simulink model "Vjezba7"  (R2016b)
settings: Solver=FixedStepAuto  StartTime=0.0  StopTime=100  FixedStep=0.0001  RelTol=1e-3
libraries: simulink_extras x3, simulink x3
settings Model: Creator=Luka  LastModifiedBy=Luka

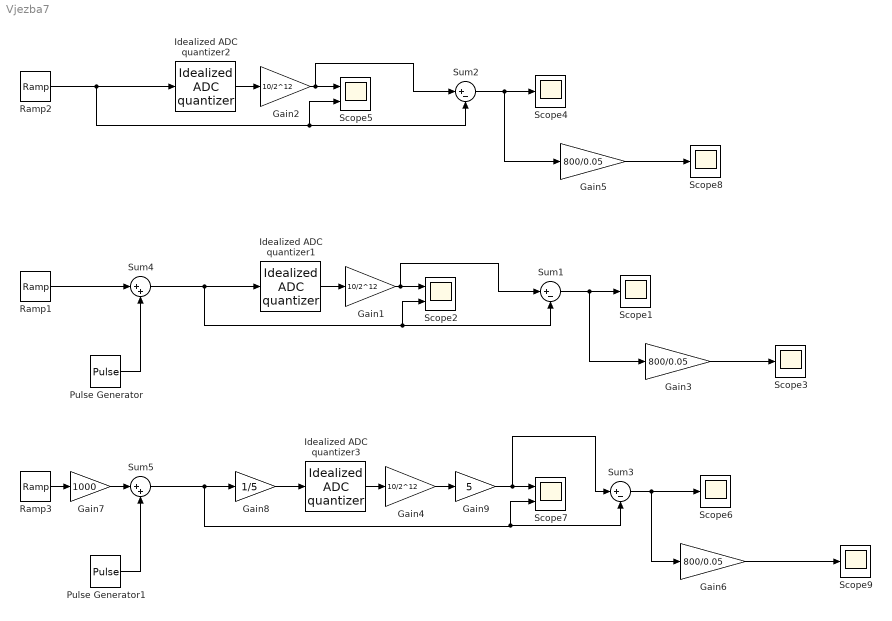
== system Vjezba7 ==
  Gain1 : Gain  Gain=10/2^12
  Gain2 : Gain  Gain=10/2^12
  Gain3 : Gain  Gain=800/0.05
  Gain4 : Gain  Gain=10/2^12
  Gain5 : Gain  Gain=800/0.05
  Gain6 : Gain  Gain=800/0.05
  Gain7 : Gain  Gain=1000
  Gain8 : Gain  Gain=1/5
  Gain9 : Gain  Gain=5
  Idealized ADC quantizer1 : simulink_extras/Additional Discrete/Idealized ADC quantizer  NumberOfConverterBits=12  Vmin=0  Vmax=10  OutputDataType=int16  OutputNegativeValues=off
  Idealized ADC quantizer2 : simulink_extras/Additional Discrete/Idealized ADC quantizer  NumberOfConverterBits=12  Vmin=0  Vmax=10  OutputDataType=int16  OutputNegativeValues=off
  Idealized ADC quantizer3 : simulink_extras/Additional Discrete/Idealized ADC quantizer  NumberOfConverterBits=12  Vmin=0  Vmax=10  OutputDataType=int16  OutputNegativeValues=off
  Pulse Generator : DiscretePulseGenerator  PulseType=Time based  Amplitude=0.01  Period=20  PulseWidth=3
  Pulse Generator1 : DiscretePulseGenerator  PulseType=Time based  Amplitude=0.01  Period=20  PulseWidth=3
  Ramp1 : simulink/Sources/Ramp  slope=0.05/800  start=0  X0=0
  Ramp2 : simulink/Sources/Ramp  slope=0.05/800  start=0  X0=0
  Ramp3 : simulink/Sources/Ramp  slope=0.05/800  start=0  X0=0
  Scope{1,3..4,6,8..9} (6 alike) : Scope
  Scope2 : Scope  NumInputPorts=2
  Scope5 : Scope  NumInputPorts=2
  Scope7 : Scope  NumInputPorts=2
  Sum1 : Sum  Inputs=|+-
  Sum2 : Sum  Inputs=|+-
  Sum3 : Sum  Inputs=|+-
  Sum4 : Sum  Inputs=|++
  Sum5 : Sum  Inputs=|++
  wires:
  Ramp2/1 -> Sum2/2, Scope5/2, Idealized ADC quantizer2/1
  Idealized ADC quantizer2/1 -> Gain2/1
  Gain2/1 -> Sum2/1, Scope5/1
  Sum2/1 -> Gain5/1, Scope4/1
  Gain5/1 -> Scope8/1
  Gain3/1 -> Scope3/1
  Sum1/1 -> Scope1/1, Gain3/1
  Gain1/1 -> Scope2/1, Sum1/1
  Idealized ADC quantizer1/1 -> Gain1/1
  Pulse Generator/1 -> Sum4/2
  Ramp1/1 -> Sum4/1
  Sum4/1 -> Scope2/2, Sum1/2, Idealized ADC quantizer1/1
  Pulse Generator1/1 -> Sum5/2
  Idealized ADC quantizer3/1 -> Gain4/1
  Sum3/1 -> Gain6/1, Scope6/1
  Gain6/1 -> Scope9/1
  Ramp3/1 -> Gain7/1
  Gain7/1 -> Sum5/1
  Gain8/1 -> Idealized ADC quantizer3/1
  Sum5/1 -> Sum3/2, Scope7/2, Gain8/1
  Gain4/1 -> Gain9/1
  Gain9/1 -> Sum3/1, Scope7/1
